simulink model "AXI_QPSK_Tx"  (R2023b)
settings: Solver=FixedStepAuto  StartTime=0.0  StopTime=10/Rb  RelTol=1e-3
PreLoadFcn:
  | Rb = 1000;   % 1kbit / s
  | Rsym = Rb/2;   % 2 bits per symbol
  | Rsymbol = Rb/2;
  | OSR = 32;
  | f_error = 120;
  | 
  | design_filters_tx
values from neighbouring files (symbols this model uses):
  CIC_fine_Tx = 2^-(CIC_right_shift - CIC_left_shift - CIC_shift_Tx)    [design_filters_tx.m]
  fCIC = fCICcomp * R_CIC    (= 25600000)    [design_filters_tx.m]
  fHB = fRRC * R_HB    (= 4000)    [design_filters_tx.m]
  R_CIC = 3200    [design_filters_tx.m]
  R_CICcomp = 2    [design_filters_tx.m]
  R_HB = 2    [design_filters_tx.m]
  R_RRC = 4    [design_filters_tx.m]
undefined symbols (not defined in the file or in its folder): AXI4, Lite
libraries: hdlBasic x309, hdlDSPIP x8, hdlsllib x2, vmcUtilities x1
(part 3 of 3)

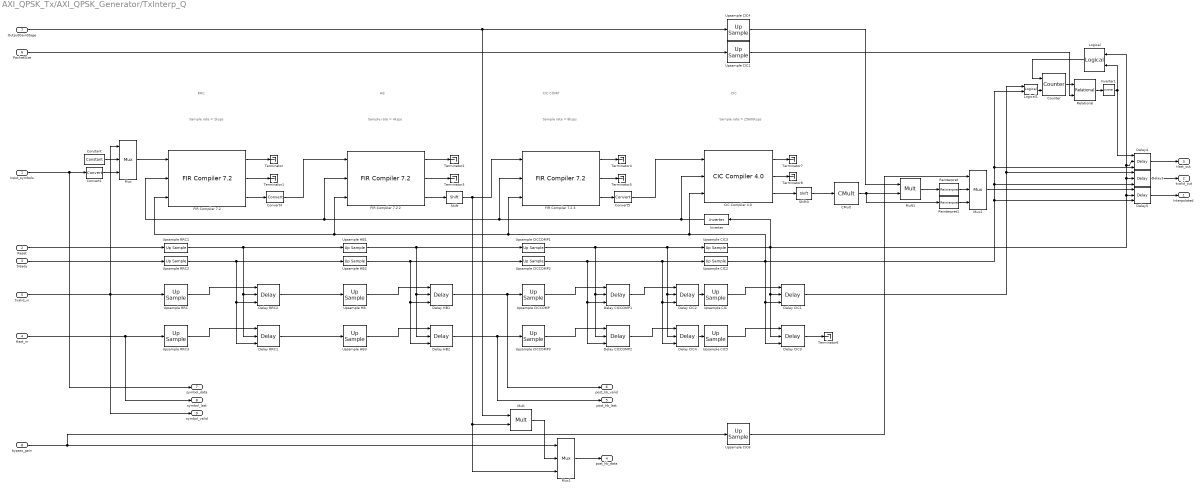
== system AXI_QPSK_Tx/AXI_QPSK_Generator/TxInterp_Q ==
  note: Sample rate
      | = 25600ksps
  note: Sample rate
      | = 8ksps
  note: Sample rate
      | = 4ksps
  note: Sample rate
      | = 2ksps
  note: CIC
  note: CIC COMP
  note: RRC
  note: HB
  Input_symbols : Inport
  Reset : Inport  Port=2
  tready : Inport  Port=3
  tlast_in : Inport  Port=4
  tvalid_in : Inport  Port=5
  PacketSize : Inport  Port=6
  OutputGainStage : Inport  Port=7
  bypass_gain : Inport  Port=8
  "CIC Compiler 4.0 " : hdlDSPIP/CIC Compiler 4.0   filter_type=Interpolation  number_of_stages=5  differential_delay=1  number_of_channels=1  sample_rate_changes=Fixed  fixed_or_initial_rate=R_CIC  minimum_rate=3200  maximum_rate=3200  ratespecification=Maximum_Possible  sampleperiod=3200  hardwareoversamplingrate=1  quantization=Full_Precision  output_data_width=65  use_xtreme_dsp_slice=on  use_streaming_interface=on  has_aclken=on  has_aresetn=on  has_dout_tready=off  trim_axipin_name=on  gui_behaviour=Sysgen_GUI  input_data_width=18  ip_name=CIC Compiler  ip_version=4.0  dsptool_ready=true  wrapper_available=true  port_translation_map={ 'aclken' => 'en', 'aresetn' => 'rst' }  ipcore_xco_need_fpga_part=true  ipcore_fpga_part=[]  ipcore_verbose=false  XmcBlockStatus=1  maskContainerNames=tabcontainer1  block_type=cic_compiler_v4_0  block_config=sysgen:rodinimport_config
  CMult : hdlBasic/CMult  const=CIC_fine_Tx  gui_display_data_type=Fixed-point  const_n_bits=16  const_bin_pt=15  float_type=Single  exp_bits=8  fraction_bits=24  en=off  latency=0  precision=User Defined  arith_type="Signed  (2's comp)"  n_bits=16  bin_pt=15  quantization=Truncate  overflow=Wrap  use_behavioral_HDL=off  mem_type=Distributed RAM  pipeline=off  XmcBlockStatus=1  maskContainerNames=tabcontainer1  block_type=cmult  block_config=sysgen:CMult_config
      settings: infoedit=[]
  Constant : hdlBasic/Constant  const=0  gui_display_data_type=Fixed-point  arith_type=Signed (2's comp)  n_bits=16  bin_pt=0  preci_type=Single  exp_width=8  frac_width=24  explicit_period=on  period=2/Rb  XmcBlockStatus=1  maskContainerNames=tabcontainer1  block_type=constant  block_config=sysgen:Constant_config
  Convert1 : hdlBasic/Convert  gui_display_data_type=Fixed-point  arith_type="Signed  (2's comp)"  n_bits=16  bin_pt=0  float_type=Single  exp_bits=8  fraction_bits=24  quantization=Truncate  overflow=Wrap  en=off  latency=0  pipeline=off  XmcBlockStatus=1  maskContainerNames=group2  block_type=convert  block_config=sysgen:Convert_config  block_width=595  block_height=885
  Convert4 : hdlBasic/Convert  gui_display_data_type=Fixed-point  arith_type="Signed  (2's comp)"  n_bits=16  bin_pt=15  float_type=Single  exp_bits=8  fraction_bits=24  quantization=Truncate  overflow=Wrap  en=off  latency=0  pipeline=off  XmcBlockStatus=1  maskContainerNames=group2  block_type=convert  block_config=sysgen:Convert_config  block_width=595  block_height=885
  Convert5 : hdlBasic/Convert  gui_display_data_type=Fixed-point  arith_type="Signed  (2's comp)"  n_bits=16  bin_pt=15  float_type=Single  exp_bits=8  fraction_bits=24  quantization=Truncate  overflow=Wrap  en=off  latency=0  pipeline=off  XmcBlockStatus=1  maskContainerNames=group2  block_type=convert  block_config=sysgen:Convert_config  block_width=595  block_height=885
  Counter : hdlBasic/Counter  cnt_type=Free running  cnt_to=Inf  operation=Up  start_count=0  cnt_by_val=1  arith_type=Unsigned  n_bits=32  bin_pt=0  load_pin=off  rst=on  en=on  explicit_period=Explicit  period=1/fCIC  use_behavioral_HDL=off  implementation=Fabric  XmcBlockStatus=1  maskContainerNames=group1  block_type=counter  block_config=sysgen:Counter_config  block_width=531  block_height=1023
  Delay CIC1 : hdlBasic/Delay  rst=on  en=on  latency=3*8  reg_retiming=off  XmcBlockStatus=1  maskContainerNames=group1  block_type=delay  block_config=sysgen:Delay_config
  Delay CIC2 : hdlBasic/Delay  rst=on  en=on  latency=4  reg_retiming=off  XmcBlockStatus=1  maskContainerNames=group1  block_type=delay  block_config=sysgen:Delay_config
  Delay CIC3 : hdlBasic/Delay  rst=on  en=on  latency=3*8-1  reg_retiming=off  XmcBlockStatus=1  maskContainerNames=group1  block_type=delay  block_config=sysgen:Delay_config
  Delay CIC4 : hdlBasic/Delay  rst=on  en=on  latency=5  reg_retiming=off  XmcBlockStatus=1  maskContainerNames=group1  block_type=delay  block_config=sysgen:Delay_config
  Delay CICCOMP1 : hdlBasic/Delay  rst=on  en=on  latency=R_CICcomp*4  reg_retiming=off  XmcBlockStatus=1  maskContainerNames=group1  block_type=delay  block_config=sysgen:Delay_config
  Delay CICCOMP2 : hdlBasic/Delay  rst=on  en=on  latency=R_CICcomp*4+1  reg_retiming=off  XmcBlockStatus=1  maskContainerNames=group1  block_type=delay  block_config=sysgen:Delay_config
  Delay HB1 : hdlBasic/Delay  rst=on  en=on  latency=R_HB*2  reg_retiming=off  XmcBlockStatus=1  maskContainerNames=group1  block_type=delay  block_config=sysgen:Delay_config
  Delay HB2 : hdlBasic/Delay  rst=on  en=on  latency=R_HB*2+1  reg_retiming=off  XmcBlockStatus=1  maskContainerNames=group1  block_type=delay  block_config=sysgen:Delay_config
  Delay RRC1 : hdlBasic/Delay  rst=on  en=on  latency=3*R_RRC  reg_retiming=off  XmcBlockStatus=1  maskContainerNames=group1  block_type=delay  block_config=sysgen:Delay_config
  Delay RRC2 : hdlBasic/Delay  rst=on  en=on  latency=R_RRC*2+1  reg_retiming=off  XmcBlockStatus=1  maskContainerNames=group1  block_type=delay  block_config=sysgen:Delay_config
  Delay3 : hdlBasic/Delay  rst=on  en=on  latency=1  reg_retiming=off  XmcBlockStatus=1  maskContainerNames=group1  block_type=delay  block_config=sysgen:Delay_config
  Delay4 : hdlBasic/Delay  rst=on  en=on  latency=1  reg_retiming=off  XmcBlockStatus=1  maskContainerNames=group1  block_type=delay  block_config=sysgen:Delay_config
  Delay5 : hdlBasic/Delay  rst=on  en=on  latency=1  reg_retiming=off  XmcBlockStatus=1  maskContainerNames=group1  block_type=delay  block_config=sysgen:Delay_config
  "FIR Compiler 7.2 " : hdlDSPIP/FIR Compiler 7.2   coefficientvector=WRRC.Numerator  coefficient_sets=1  coefficient_reload=off  filter_type=Interpolation  rate_change_type=Integer  interpolation_rate=R_RRC  decimation_rate=1  zero_pack_factor=1  channel_sequence=Basic  number_channels=1  pattern_list='P4-0,P4-1,P4-2,P4-3,P4-4'  number_paths=1  ratespecification=Maximum_Possible  sampleperiod=1  hardwareoversamplingrate=1  coefficient_sign=Signed  quantization=Quantize_Only  coefficient_width=16  bestprecision=on  coefficient_fractional_bits=15  coefficient_structure=Inferred  output_rounding_mode=Full_Precision  output_width=31  filter_architecture=Systolic_Multiply_Accumulate  optimization_goal=Area  optimization_list='None'  data_buffer_type=Automatic  coefficient_buffer_type=Automatic  input_buffer_type=Automatic  output_buffer_type=Automatic  preference_for_other_storage=Automatic  multi_column_support=Automatic  columnconfig='13'  inter_column_pipe_length=4  data_has_tlast=Not_Required  m_data_has_tready=off  s_data_has_fifo=off  s_data_has_tuser=Not_Required  m_data_has_tuser=Not_Required  s_config_sync_mode=On_Vector  s_config_method=Single  num_reload_slots=1  has_aclken=on  has_aresetn=on  reset_data_vector=on  trim_axipin_name=on  simulation_type=hybrid_sim  simulation_model=sysgen:xfirv7_2_cmodel  data_path_portlist={ 's_axis_data_tdata', 'm_axis_data_tdata' }  passband_min=0.0  passband_max=0.5  stopband_min=0.5  stopband_max=1.0  filter_selection=1  gui_behaviour='Sysgen_GUI'  data_sign=Signed  data_width=16  data_fractional_bits=0  data_tuser_width=1  wrapper_available=true  ip_wrap_arbitrary_binary_point=true  ip_name=FIR Compiler  ip_version=7.2  dsptool_ready=true  ipcore_usecache=true  ipcore_useipmodelcache=true  port_translation_map={ 'aclken' => 'en', 'aresetn' => 'rst' }  run_core_at_system_period=true  ipcore_xco_need_fpga_part=true  ipcore_fpga_part=[]  XmcBlockStatus=1  maskContainerNames=tabcontainer1  block_type=fir_compiler_v7_2  block_config=sysgen:rodinimport_config  block_width=820  block_height=600
  FIR Compiler 7.2 2 : hdlDSPIP/FIR Compiler 7.2   coefficientvector=HB.Numerator  coefficient_sets=1  coefficient_reload=off  filter_type=Interpolation  rate_change_type=Integer  interpolation_rate=2  decimation_rate=1  zero_pack_factor=1  channel_sequence=Basic  number_channels=1  pattern_list='P4-0,P4-1,P4-2,P4-3,P4-4'  number_paths=1  ratespecification=Maximum_Possible  sampleperiod=1  hardwareoversamplingrate=1  coefficient_sign=Signed  quantization=Quantize_Only  coefficient_width=16  bestprecision=on  coefficient_fractional_bits=15  coefficient_structure=Inferred  output_rounding_mode=Full_Precision  output_width=32  filter_architecture=Systolic_Multiply_Accumulate  optimization_goal=Area  optimization_list='None'  data_buffer_type=Automatic  coefficient_buffer_type=Automatic  input_buffer_type=Automatic  output_buffer_type=Automatic  preference_for_other_storage=Automatic  multi_column_support=Automatic  columnconfig='6'  inter_column_pipe_length=4  data_has_tlast=Not_Required  m_data_has_tready=off  s_data_has_fifo=off  s_data_has_tuser=Not_Required  m_data_has_tuser=Not_Required  s_config_sync_mode=On_Vector  s_config_method=Single  num_reload_slots=1  has_aclken=on  has_aresetn=on  reset_data_vector=on  trim_axipin_name=on  simulation_type=hybrid_sim  simulation_model=sysgen:xfirv7_2_cmodel  data_path_portlist={ 's_axis_data_tdata', 'm_axis_data_tdata' }  passband_min=0.0  passband_max=0.5  stopband_min=0.5  stopband_max=1.0  filter_selection=1  gui_behaviour='Sysgen_GUI'  data_sign=Signed  data_width=16  data_fractional_bits=0  data_tuser_width=1  wrapper_available=true  ip_wrap_arbitrary_binary_point=true  ip_name=FIR Compiler  ip_version=7.2  dsptool_ready=true  ipcore_usecache=true  ipcore_useipmodelcache=true  port_translation_map={ 'aclken' => 'en', 'aresetn' => 'rst' }  run_core_at_system_period=true  ipcore_xco_need_fpga_part=true  ipcore_fpga_part=[]  XmcBlockStatus=1  maskContainerNames=tabcontainer1  block_type=fir_compiler_v7_2  block_config=sysgen:rodinimport_config  block_width=820  block_height=600
  FIR Compiler 7.2 3 : hdlDSPIP/FIR Compiler 7.2   coefficientvector=WComp.Numerator  coefficient_sets=1  coefficient_reload=off  filter_type=Interpolation  rate_change_type=Integer  interpolation_rate=R_CICcomp  decimation_rate=1  zero_pack_factor=1  channel_sequence=Basic  number_channels=1  pattern_list='P4-0,P4-1,P4-2,P4-3,P4-4'  number_paths=1  ratespecification=Maximum_Possible  sampleperiod=1  hardwareoversamplingrate=1  coefficient_sign=Signed  quantization=Quantize_Only  coefficient_width=16  bestprecision=on  coefficient_fractional_bits=15  coefficient_structure=Inferred  output_rounding_mode=Full_Precision  output_width=33  filter_architecture=Systolic_Multiply_Accumulate  optimization_goal=Area  optimization_list='None'  data_buffer_type=Automatic  coefficient_buffer_type=Automatic  input_buffer_type=Automatic  output_buffer_type=Automatic  preference_for_other_storage=Automatic  multi_column_support=Automatic  columnconfig='19'  inter_column_pipe_length=4  data_has_tlast=Not_Required  m_data_has_tready=off  s_data_has_fifo=off  s_data_has_tuser=Not_Required  m_data_has_tuser=Not_Required  s_config_sync_mode=On_Vector  s_config_method=Single  num_reload_slots=1  has_aclken=on  has_aresetn=on  reset_data_vector=on  trim_axipin_name=on  simulation_type=hybrid_sim  simulation_model=sysgen:xfirv7_2_cmodel  data_path_portlist={ 's_axis_data_tdata', 'm_axis_data_tdata' }  passband_min=0.0  passband_max=0.5  stopband_min=0.5  stopband_max=1.0  filter_selection=1  gui_behaviour='Sysgen_GUI'  data_sign=Signed  data_width=16  data_fractional_bits=0  data_tuser_width=1  wrapper_available=true  ip_wrap_arbitrary_binary_point=true  ip_name=FIR Compiler  ip_version=7.2  dsptool_ready=true  ipcore_usecache=true  ipcore_useipmodelcache=true  port_translation_map={ 'aclken' => 'en', 'aresetn' => 'rst' }  run_core_at_system_period=true  ipcore_xco_need_fpga_part=true  ipcore_fpga_part=[]  XmcBlockStatus=1  maskContainerNames=tabcontainer1  block_type=fir_compiler_v7_2  block_config=sysgen:rodinimport_config  block_width=820  block_height=600
  Inverter : hdlBasic/Inverter  en=off  latency=0  XmcBlockStatus=1  maskContainerNames=group2  block_type=inv  block_config=sysgen:Inverter_config
  Inverter1 : hdlBasic/Inverter  en=off  latency=0  XmcBlockStatus=1  maskContainerNames=group2  block_type=inv  block_config=sysgen:Inverter_config
  Logical : hdlBasic/Logical  logical_function=OR  inputs=2  en=off  latency=0  precision=Full  arith_type=Unsigned  n_bits=16  bin_pt=0  align_bp=on  overflow=[]  quantization=[]  XmcBlockStatus=1  maskContainerNames=tabcontainer1  block_type=logical  block_config=sysgen:Logical_config
  Logical1 : hdlBasic/Logical  logical_function=AND  inputs=2  en=off  latency=0  precision=Full  arith_type=Unsigned  n_bits=16  bin_pt=0  align_bp=on  overflow=[]  quantization=[]  XmcBlockStatus=1  maskContainerNames=tabcontainer1  block_type=logical  block_config=sysgen:Logical_config
  Mult : hdlBasic/Mult  precision=User Defined  arith_type="Signed  (2's comp)"  n_bits=16  bin_pt=15  quantization=Truncate  overflow=Wrap  en=off  latency=0  use_behavioral_HDL=off  opt=Speed  use_embedded=on  optimum_pipeline=off  pipeline=on  use_rpm=on  placement_style=Triangular  XmcBlockStatus=1  maskContainerNames=group1  block_type=mult  block_config=sysgen:Mult_config  block_width=598  block_height=876
  Mult1 : hdlBasic/Mult  precision=User Defined  arith_type="Signed  (2's comp)"  n_bits=16  bin_pt=15  quantization=Truncate  overflow=Wrap  en=off  latency=0  use_behavioral_HDL=off  opt=Speed  use_embedded=on  optimum_pipeline=off  pipeline=on  use_rpm=on  placement_style=Triangular  XmcBlockStatus=1  maskContainerNames=group1  block_type=mult  block_config=sysgen:Mult_config  block_width=598  block_height=876
  Mux : hdlBasic/Mux  inputs=2  en=off  latency=0  precision=Full  arith_type=Unsigned  n_bits=16  bin_pt=14  quantization=Truncate  overflow=Wrap  XmcBlockStatus=1  maskContainerNames=tabcontainer1  block_type=mux  block_config=sysgen:Mux_config
  Mux1 : hdlBasic/Mux  inputs=2  en=off  latency=0  precision=Full  arith_type=Unsigned  n_bits=16  bin_pt=14  quantization=Truncate  overflow=Wrap  XmcBlockStatus=1  maskContainerNames=tabcontainer1  block_type=mux  block_config=sysgen:Mux_config
  Mux2 : hdlBasic/Mux  inputs=2  en=off  latency=0  precision=Full  arith_type=Unsigned  n_bits=16  bin_pt=14  quantization=Truncate  overflow=Wrap  XmcBlockStatus=1  maskContainerNames=tabcontainer1  block_type=mux  block_config=sysgen:Mux_config
  Reinterpret : hdlBasic/Reinterpret  force_arith_type=on  arith_type=Unsigned  force_bin_pt=on  bin_pt=0  XmcBlockStatus=1  maskContainerNames=group1  block_type=reinterpret  block_config=sysgen:Reinterpret_config
  Reinterpret1 : hdlBasic/Reinterpret  force_arith_type=on  arith_type=Unsigned  force_bin_pt=on  bin_pt=0  XmcBlockStatus=1  maskContainerNames=group1  block_type=reinterpret  block_config=sysgen:Reinterpret_config
  Relational : hdlBasic/Relational  mode=a<b  op_type=Bool  en=off  latency=0  XmcBlockStatus=1  maskContainerNames=tabcontainer1  block_type=relational  block_config=sysgen:Relational_config
  Shift : hdlBasic/Shift  shift_dir=Left  shift_bits=1  en=off  latency=0  precision=User Defined  arith_type="Signed  (2's comp)"  n_bits=16  bin_pt=15  quantization=Truncate  overflow=Wrap  XmcBlockStatus=1  maskContainerNames=group2  block_type=shift  block_config=sysgen:Shift_config
  Shift3 : hdlBasic/Shift  shift_dir=Right  shift_bits=CIC_shift_Tx  en=off  latency=0  precision=User Defined  arith_type="Signed  (2's comp)"  n_bits=17  bin_pt=14  quantization=Truncate  overflow=Wrap  XmcBlockStatus=1  maskContainerNames=group2  block_type=shift  block_config=sysgen:Shift_config
  Terminator{,1..8} (9 alike) : Terminator
  Upsample CIC : hdlBasic/Up Sample  sample_ratio=R_CIC  copy_samples=on  en=off  latency=0  XmcBlockStatus=1  maskContainerNames=group1  block_type=usamp  block_config=sysgen:Upsample_config
  Upsample CIC1 : hdlBasic/Up Sample  sample_ratio=fCIC/(Rb/2)  copy_samples=on  en=off  latency=0  XmcBlockStatus=1  maskContainerNames=group1  block_type=usamp  block_config=sysgen:Upsample_config
  Upsample CIC2 : hdlBasic/Up Sample  sample_ratio=R_CIC  copy_samples=on  en=off  latency=0  XmcBlockStatus=1  maskContainerNames=group1  block_type=usamp  block_config=sysgen:Upsample_config
  Upsample CIC3 : hdlBasic/Up Sample  sample_ratio=R_CIC  copy_samples=on  en=off  latency=0  XmcBlockStatus=1  maskContainerNames=group1  block_type=usamp  block_config=sysgen:Upsample_config
  Upsample CIC4 : hdlBasic/Up Sample  sample_ratio=fCIC/fHB  copy_samples=on  en=off  latency=0  XmcBlockStatus=1  maskContainerNames=group1  block_type=usamp  block_config=sysgen:Upsample_config
  Upsample CIC5 : hdlBasic/Up Sample  sample_ratio=R_CIC  copy_samples=off  en=off  latency=0  XmcBlockStatus=1  maskContainerNames=group1  block_type=usamp  block_config=sysgen:Upsample_config
  Upsample CIC6 : hdlBasic/Up Sample  sample_ratio=fCIC/fHB  copy_samples=on  en=off  latency=0  XmcBlockStatus=1  maskContainerNames=group1  block_type=usamp  block_config=sysgen:Upsample_config
  Upsample CICCOMP : hdlBasic/Up Sample  sample_ratio=R_CICcomp  copy_samples=on  en=off  latency=0  XmcBlockStatus=1  maskContainerNames=group1  block_type=usamp  block_config=sysgen:Upsample_config
  Upsample CICCOMP1 : hdlBasic/Up Sample  sample_ratio=R_CICcomp  copy_samples=on  en=off  latency=0  XmcBlockStatus=1  maskContainerNames=group1  block_type=usamp  block_config=sysgen:Upsample_config
  Upsample CICCOMP2 : hdlBasic/Up Sample  sample_ratio=R_CICcomp  copy_samples=on  en=off  latency=0  XmcBlockStatus=1  maskContainerNames=group1  block_type=usamp  block_config=sysgen:Upsample_config
  Upsample CICCOMP3 : hdlBasic/Up Sample  sample_ratio=R_CICcomp  copy_samples=off  en=off  latency=0  XmcBlockStatus=1  maskContainerNames=group1  block_type=usamp  block_config=sysgen:Upsample_config
  Upsample HB : hdlBasic/Up Sample  sample_ratio=R_HB  copy_samples=on  en=off  latency=0  XmcBlockStatus=1  maskContainerNames=group1  block_type=usamp  block_config=sysgen:Upsample_config
  Upsample HB1 : hdlBasic/Up Sample  sample_ratio=R_HB  copy_samples=on  en=off  latency=0  XmcBlockStatus=1  maskContainerNames=group1  block_type=usamp  block_config=sysgen:Upsample_config
  Upsample HB2 : hdlBasic/Up Sample  sample_ratio=R_HB  copy_samples=on  en=off  latency=0  XmcBlockStatus=1  maskContainerNames=group1  block_type=usamp  block_config=sysgen:Upsample_config
  Upsample HB3 : hdlBasic/Up Sample  sample_ratio=R_HB  copy_samples=off  en=off  latency=0  XmcBlockStatus=1  maskContainerNames=group1  block_type=usamp  block_config=sysgen:Upsample_config
  Upsample RRC : hdlBasic/Up Sample  sample_ratio=R_RRC  copy_samples=on  en=off  latency=0  XmcBlockStatus=1  maskContainerNames=group1  block_type=usamp  block_config=sysgen:Upsample_config
  Upsample RRC1 : hdlBasic/Up Sample  sample_ratio=R_RRC  copy_samples=on  en=off  latency=0  XmcBlockStatus=1  maskContainerNames=group1  block_type=usamp  block_config=sysgen:Upsample_config
  Upsample RRC2 : hdlBasic/Up Sample  sample_ratio=R_RRC  copy_samples=on  en=off  latency=0  XmcBlockStatus=1  maskContainerNames=group1  block_type=usamp  block_config=sysgen:Upsample_config
  Upsample RRC3 : hdlBasic/Up Sample  sample_ratio=R_RRC  copy_samples=off  en=off  latency=0  XmcBlockStatus=1  maskContainerNames=group1  block_type=usamp  block_config=sysgen:Upsample_config
  Interpolated : Outport  VectorParamsAs1DForOutWhenUnconnected=off
  tvalid_out : Outport  Port=2  VectorParamsAs1DForOutWhenUnconnected=off
  tlast_out : Outport  Port=3  VectorParamsAs1DForOutWhenUnconnected=off
  post_hb_data : Outport  Port=4  VectorParamsAs1DForOutWhenUnconnected=off
  post_hb_last : Outport  Port=5  VectorParamsAs1DForOutWhenUnconnected=off
  post_hb_valid : Outport  Port=6  VectorParamsAs1DForOutWhenUnconnected=off
  symbol_data : Outport  Port=7  VectorParamsAs1DForOutWhenUnconnected=off
  symbol_last : Outport  Port=8  VectorParamsAs1DForOutWhenUnconnected=off
  symbol_valid : Outport  Port=9  VectorParamsAs1DForOutWhenUnconnected=off
  wires:
  Mult/1 -> Mux1/2
  Mux1/1 -> post_hb_data/1
  Upsample CIC4/1 -> Mult1/1
  Mult1/1 -> Reinterpret/1
  Delay CIC3/1 -> Terminator6/1
  Delay HB1/1 -> Upsample CICCOMP/1, post_hb_valid/1
  Delay HB2/1 -> post_hb_last/1, Upsample CICCOMP3/1
  Constant/1 -> Mux/2
  Input_symbols/1 -> symbol_data/1, Convert1/1
  Mux/1 -> "FIR Compiler 7.2 "/1
  Delay CICCOMP2/1 -> Delay CIC4/1
  Delay CIC4/1 -> Upsample CIC5/1
  Delay CICCOMP1/1 -> Delay CIC2/1
  Delay CIC2/1 -> Upsample CIC/1
  Inverter/1 -> "CIC Compiler 4.0 "/2, FIR Compiler 7.2 2/2, "FIR Compiler 7.2 "/2, FIR Compiler 7.2 3/2
  Upsample CIC5/1 -> Delay CIC3/1
  Upsample RRC1/1 -> Upsample HB1/1, Delay RRC2/2, Delay RRC1/2
  Upsample RRC2/1 -> Upsample HB2/1, Delay RRC2/3, Delay RRC1/3
  Upsample HB1/1 -> Upsample CICCOMP1/1, Delay HB1/2, Delay HB2/2
  Upsample HB2/1 -> Upsample CICCOMP2/1, Delay HB1/3, Delay HB2/3
  Upsample CICCOMP1/1 -> Upsample CIC3/1, Delay CIC2/2, Delay CIC4/2, Delay CICCOMP1/2, Delay CICCOMP2/2
  Upsample CICCOMP2/1 -> Upsample CIC2/1, Delay CIC2/3, Delay CIC4/3, Delay CICCOMP1/3, Delay CICCOMP2/3
  tlast_in/1 -> symbol_last/1, Upsample RRC3/1
  Delay RRC1/1 -> Upsample HB3/1
  Upsample RRC3/1 -> Delay RRC1/1
  Upsample HB3/1 -> Delay HB2/1
  Upsample CICCOMP3/1 -> Delay CICCOMP2/1
  tready/1 -> Upsample RRC2/1
  Delay CIC1/1 -> Delay3/1, Logical1/1
  Upsample CICCOMP/1 -> Delay CICCOMP1/1
  Upsample HB/1 -> Delay HB1/1
  Upsample RRC/1 -> Delay RRC2/1
  Delay RRC2/1 -> Upsample HB/1
  tvalid_in/1 -> Mux/1, symbol_valid/1, Upsample RRC/1
  Upsample CIC3/1 -> Inverter/1, Delay4/2, Logical/1, Delay3/2, Delay5/2, Delay CIC1/2, Delay CIC3/2
  Upsample CIC2/1 -> "CIC Compiler 4.0 "/3, FIR Compiler 7.2 3/3, FIR Compiler 7.2 2/3, "FIR Compiler 7.2 "/3, Delay5/3, Delay3/3, Delay4/3, Logical1/2, Delay CIC1/3, Delay CIC3/3
  "CIC Compiler 4.0 "/2 -> Terminator8/1
  Upsample CIC/1 -> Delay CIC1/1
  Reset/1 -> Upsample RRC1/1
  Convert5/1 -> "CIC Compiler 4.0 "/1
  "CIC Compiler 4.0 "/1 -> Terminator7/1
  FIR Compiler 7.2 3/2 -> Terminator5/1
  FIR Compiler 7.2 3/1 -> Terminator4/1
  FIR Compiler 7.2 3/3 -> Convert5/1
  FIR Compiler 7.2 2/1 -> Terminator2/1
  FIR Compiler 7.2 2/2 -> Terminator3/1
  FIR Compiler 7.2 2/3 -> Shift/1
  "FIR Compiler 7.2 "/3 -> Convert4/1
  Shift3/1 -> CMult/1
  "FIR Compiler 7.2 "/2 -> Terminator1/1
  "FIR Compiler 7.2 "/1 -> Terminator/1
  PacketSize/1 -> Upsample CIC1/1
  Upsample CIC1/1 -> Relational/2
  Counter/1 -> Relational/1
  Logical/1 -> Counter/1
  Inverter1/1 -> Delay4/1, Logical/2
  Relational/1 -> Inverter1/1
  Delay4/1 -> tlast_out/1
  Delay3/1 -> tvalid_out/1
  Delay5/1 -> Interpolated/1
  Logical1/1 -> Counter/2
  "CIC Compiler 4.0 "/3 -> Shift3/1
  Convert4/1 -> FIR Compiler 7.2 2/1
  Convert1/1 -> Mux/3
  Shift/1 -> FIR Compiler 7.2 3/1, Mult/2, Mux1/3
  CMult/1 -> Mult1/2, Reinterpret1/1
  OutputGainStage/1 -> Upsample CIC4/1, Mult/1
  Reinterpret/1 -> Mux2/2
  Mux2/1 -> Delay5/1
  Reinterpret1/1 -> Mux2/3
  bypass_gain/1 -> Upsample CIC6/1, Mux1/1
  Upsample CIC6/1 -> Mux2/1

== system AXI_QPSK_Tx/AXI_QPSK_Generator/PostHB_Time_Domain/M_AXIS_SYMBOL_CTRL ==
  i_data : Inport
  tvalid_in : Inport  Port=2
  q_data : Inport  Port=3
  reset : Inport  Port=4
  packet_size : Inport  Port=5
  tready_in : Inport  Port=6
  transfer : Inport  Port=7
  auto_restart : Inport  Port=8
  AXI_Write_Interface : Subsystem
  Concat : hdlBasic/Concat  num_inputs=2  XmcBlockStatus=1  maskContainerNames=group1  block_type=concat  block_config=sysgen:Concat_config
  Reinterpret : hdlBasic/Reinterpret  force_arith_type=on  arith_type=Unsigned  force_bin_pt=on  bin_pt=0  XmcBlockStatus=1  maskContainerNames=group1  block_type=reinterpret  block_config=sysgen:Reinterpret_config
  Reinterpret1 : hdlBasic/Reinterpret  force_arith_type=on  arith_type=Unsigned  force_bin_pt=on  bin_pt=0  XmcBlockStatus=1  maskContainerNames=group1  block_type=reinterpret  block_config=sysgen:Reinterpret_config
  tdata_out : Outport  VectorParamsAs1DForOutWhenUnconnected=off
  tvalid_out : Outport  Port=2  VectorParamsAs1DForOutWhenUnconnected=off
  tlast_out : Outport  Port=3  VectorParamsAs1DForOutWhenUnconnected=off
  wires:
  AXI_Write_Interface/1(tdata_out) -> tdata_out/1
  AXI_Write_Interface/3(tvalid_out) -> tvalid_out/1
  AXI_Write_Interface/2(tlast_out) -> tlast_out/1
  tready_in/1 -> AXI_Write_Interface/7(tready)
  auto_restart/1 -> AXI_Write_Interface/3(auto_restart)
  transfer/1 -> AXI_Write_Interface/2(transfer)
  Concat/1 -> AXI_Write_Interface/5(tdata_in)
  reset/1 -> AXI_Write_Interface/1(int_reset)
  tvalid_in/1 -> AXI_Write_Interface/6(tvalid_in)
  packet_size/1 -> AXI_Write_Interface/4(packet_size)
  Reinterpret/1 -> Concat/1
  Reinterpret1/1 -> Concat/2
  q_data/1 -> Reinterpret/1
  i_data/1 -> Reinterpret1/1

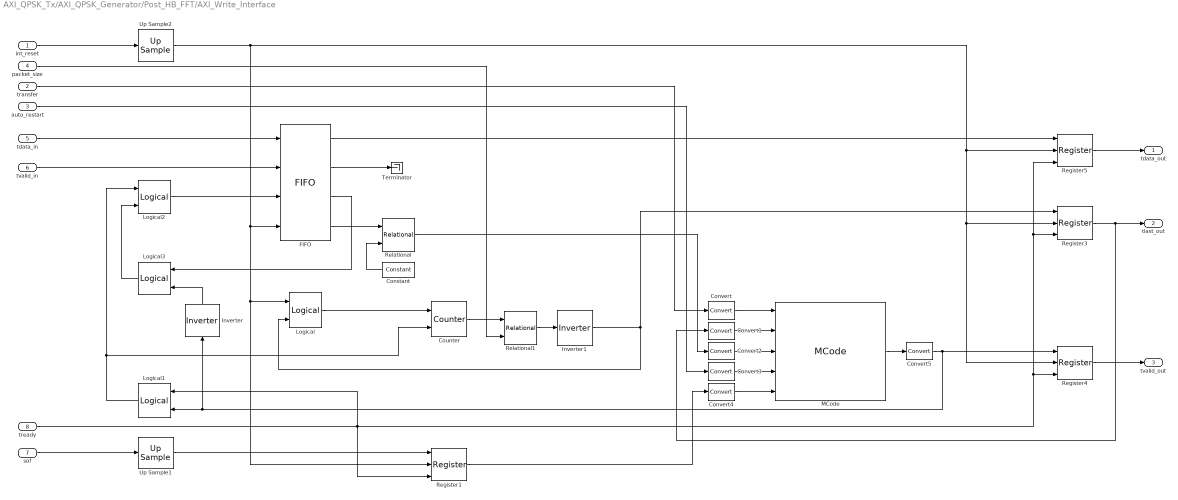
== system AXI_QPSK_Tx/AXI_QPSK_Generator/Post_HB_FFT/AXI_Write_Interface ==
  int_reset : Inport
  transfer : Inport  Port=2
  auto_restart : Inport  Port=3
  packet_size : Inport  Port=4
  tdata_in : Inport  Port=5
  tvalid_in : Inport  Port=6
  sof : Inport  Port=7
  tready : Inport  Port=8
  Constant : hdlBasic/Constant  const=8192/2-1  gui_display_data_type=Fixed-point  arith_type=Unsigned  n_bits=13  bin_pt=0  preci_type=Single  exp_width=8  frac_width=24  explicit_period=on  period=1/fCIC  XmcBlockStatus=1  maskContainerNames=tabcontainer1  block_type=constant  block_config=sysgen:Constant_config
  Convert{,1..4} (5 alike) : hdlBasic/Convert  gui_display_data_type=Fixed-point  arith_type=Unsigned  n_bits=1  bin_pt=0  float_type=Single  exp_bits=8  fraction_bits=24  quantization=Truncate  overflow=Wrap  en=off  latency=0  pipeline=off  XmcBlockStatus=1  maskContainerNames=group2  block_type=convert  block_config=sysgen:Convert_config  block_width=595  block_height=885
  Convert5 : hdlBasic/Convert  gui_display_data_type=Boolean  arith_type=Boolean  n_bits=1  bin_pt=0  float_type=Single  exp_bits=8  fraction_bits=24  quantization=Truncate  overflow=Wrap  en=off  latency=0  pipeline=off  XmcBlockStatus=1  maskContainerNames=group2  block_type=convert  block_config=sysgen:Convert_config  block_width=595  block_height=885
  Counter : hdlBasic/Counter  cnt_type=Free running  cnt_to=Inf  operation=Up  start_count=0  cnt_by_val=1  arith_type=Unsigned  n_bits=32  bin_pt=0  load_pin=off  rst=on  en=on  explicit_period=Explicit  period=1/fCIC  use_behavioral_HDL=off  implementation=Fabric  XmcBlockStatus=1  maskContainerNames=group1  block_type=counter  block_config=sysgen:Counter_config  block_width=531  block_height=1023
  FIFO : hdlBasic/FIFO  mem_type=Block RAM  performance_options=Standard_FIFO  embedded_registers=off  depth=8K  use_asym_data_widths=off  asym_read_width=32  percent_nbits=1  rst=on  rst_latency=2  en=off  use_dcount=on  use_percent_full_port=off  use_almost_empty=off  almost_empty_thresh=2  use_almost_full=off  use_rd_rst_busy=off  use_wr_rst_busy=off  almost_full_thresh=14  almost_empty_offset=[]  almost_full_offset=[]  explicit_period=off  period=[]  store_only_valid=[]  init_zero=[]  simulation_type=fast_sim  XmcBlockStatus=1  maskContainerNames=tabcontainer1  block_type=fifo  block_config=sysgen:FIFO_config  block_width=538  block_height=997
      settings: infoedit=[]
  Inverter : hdlBasic/Inverter  en=off  latency=0  XmcBlockStatus=1  maskContainerNames=group2  block_type=inv  block_config=sysgen:Inverter_config
  Inverter1 : hdlBasic/Inverter  en=off  latency=0  XmcBlockStatus=1  maskContainerNames=group2  block_type=inv  block_config=sysgen:Inverter_config
  Logical : hdlBasic/Logical  logical_function=OR  inputs=2  en=off  latency=0  precision=Full  arith_type=Unsigned  n_bits=16  bin_pt=0  align_bp=on  overflow=[]  quantization=[]  XmcBlockStatus=1  maskContainerNames=tabcontainer1  block_type=logical  block_config=sysgen:Logical_config
  Logical1 : hdlBasic/Logical  logical_function=AND  inputs=2  en=off  latency=0  precision=Full  arith_type=Unsigned  n_bits=16  bin_pt=0  align_bp=on  overflow=[]  quantization=[]  XmcBlockStatus=1  maskContainerNames=tabcontainer1  block_type=logical  block_config=sysgen:Logical_config
  Logical2 : hdlBasic/Logical  logical_function=OR  inputs=2  en=off  latency=0  precision=Full  arith_type=Unsigned  n_bits=16  bin_pt=0  align_bp=on  overflow=[]  quantization=[]  XmcBlockStatus=1  maskContainerNames=tabcontainer1  block_type=logical  block_config=sysgen:Logical_config
  Logical3 : hdlBasic/Logical  logical_function=AND  inputs=2  en=off  latency=0  precision=Full  arith_type=Unsigned  n_bits=16  bin_pt=0  align_bp=on  overflow=[]  quantization=[]  XmcBlockStatus=1  maskContainerNames=tabcontainer1  block_type=logical  block_config=sysgen:Logical_config
  MCode : hdlBasic/MCode  mfname=CtrlFSM_FFT_MOD  explicit_period=on  period=1/fCIC  iptable={'AXIwrite','';'tlast','';'dcount','';'AXIauto','';'sof',''}  optable={'re','off'}  enable_stdout=off  enable_debug=off  suppress_output=on  defparams={}  hide_port_list={}  block_type=mcode  block_width=444  block_height=788
      settings: infoedit=Pass input values to a MATLAB function for evaluation in Xilinx fixed-point type. The input ports of the block are input arguments of the function. The output ports of the block are output arguments of the function.
  Register{1,3..5} (4 alike) : hdlBasic/Register  init=0  rst=on  en=on  XmcBlockStatus=1  maskContainerNames=tabcontainer1  block_type=register  block_config=sysgen:Register_config
  Relational : hdlBasic/Relational  mode=a>=b  op_type=Bool  en=off  latency=0  XmcBlockStatus=1  maskContainerNames=tabcontainer1  block_type=relational  block_config=sysgen:Relational_config
  Relational1 : hdlBasic/Relational  mode=a<b  op_type=Bool  en=off  latency=0  XmcBlockStatus=1  maskContainerNames=tabcontainer1  block_type=relational  block_config=sysgen:Relational_config
  Terminator : Terminator
  Up Sample1 : hdlBasic/Up Sample  sample_ratio=fCIC/(fHB)  copy_samples=off  en=off  latency=0  XmcBlockStatus=1  maskContainerNames=group1  block_type=usamp  block_config=sysgen:Upsample_config
  Up Sample2 : hdlBasic/Up Sample  sample_ratio=fCIC/(fHB)  copy_samples=off  en=off  latency=0  XmcBlockStatus=1  maskContainerNames=group1  block_type=usamp  block_config=sysgen:Upsample_config
  tdata_out : Outport  VectorParamsAs1DForOutWhenUnconnected=off
  tlast_out : Outport  Port=2  VectorParamsAs1DForOutWhenUnconnected=off
  tvalid_out : Outport  Port=3  VectorParamsAs1DForOutWhenUnconnected=off
  wires:
  Up Sample1/1 -> Register1/1
  Register1/1 -> Convert4/1
  sof/1 -> Up Sample1/1
  Convert4/1 -> MCode/5
  tvalid_in/1 -> FIFO/2
  FIFO/1 -> Register5/1
  Register5/1 -> tdata_out/1
  Convert5/1 -> Logical1/2, Inverter/1, Register4/1
  Register4/1 -> tvalid_out/1
  Register3/1 -> tlast_out/1, Convert1/1
  FIFO/4 -> Relational/1
  auto_restart/1 -> Convert3/1
  Logical3/1 -> Logical2/2
  MCode/1 -> Convert5/1
  packet_size/1 -> Relational1/2
  Constant/1 -> Relational/2
  Relational/1 -> Convert2/1
  Logical/1 -> Counter/1
  Counter/1 -> Relational1/1
  Relational1/1 -> Inverter1/1
  FIFO/3 -> Logical3/1
  tdata_in/1 -> FIFO/1
  Logical1/1 -> Counter/2, Logical2/1
  Inverter1/1 -> Register3/1, Logical/2
  Convert2/1 -> MCode/3
  Convert3/1 -> MCode/4
  tready/1 -> Logical1/1, Register4/3, Register5/3, Register3/3, Register1/3
  Inverter/1 -> Logical3/2
  int_reset/1 -> Up Sample2/1
  transfer/1 -> Convert/1
  Convert/1 -> MCode/1
  Convert1/1 -> MCode/2
  Logical2/1 -> FIFO/3
  FIFO/2 -> Terminator/1
  Up Sample2/1 -> Register4/2, Register3/2, Register5/2, FIFO/4, Logical/1, Register1/2

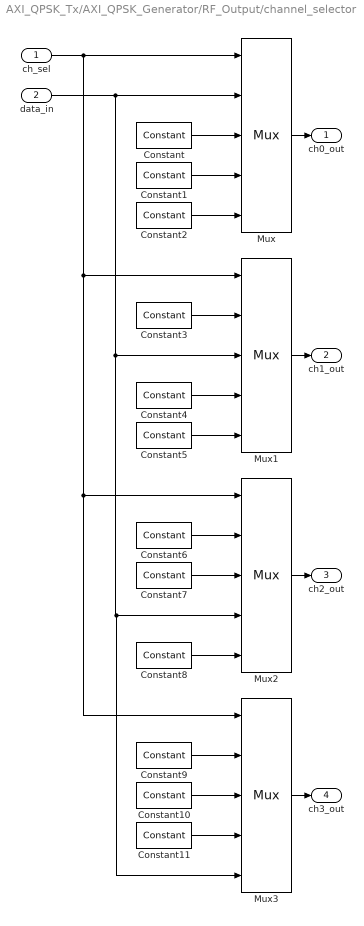
== system AXI_QPSK_Tx/AXI_QPSK_Generator/RF_Output/channel_selector ==
  ch_sel : Inport
  data_in : Inport  Port=2
  Constant{,1..11} (12 alike) : hdlBasic/Constant  const=0  gui_display_data_type=Fixed-point  arith_type=Unsigned  n_bits=32  bin_pt=0  preci_type=Single  exp_width=8  frac_width=24  explicit_period=off  period=1  XmcBlockStatus=1  maskContainerNames=tabcontainer1  block_type=constant  block_config=sysgen:Constant_config
  Mux{,1..3} (4 alike) : hdlBasic/Mux  inputs=4  en=off  latency=1  precision=Full  arith_type=Unsigned  n_bits=16  bin_pt=14  quantization=Truncate  overflow=Wrap  XmcBlockStatus=1  maskContainerNames=tabcontainer1  block_type=mux  block_config=sysgen:Mux_config
  ch0_out : Outport
  ch1_out : Outport  Port=2
  ch2_out : Outport  Port=3
  ch3_out : Outport  Port=4
  wires:
  Constant2/1 -> Mux/5
  Constant7/1 -> Mux2/3
  Constant1/1 -> Mux/4
  Constant11/1 -> Mux3/4
  Constant4/1 -> Mux1/4
  Constant6/1 -> Mux2/2
  Constant/1 -> Mux/3
  Constant5/1 -> Mux1/5
  Constant3/1 -> Mux1/2
  Constant8/1 -> Mux2/5
  Constant10/1 -> Mux3/3
  Constant9/1 -> Mux3/2
  data_in/1 -> Mux3/5, Mux2/4, Mux1/3, Mux/2
  ch_sel/1 -> Mux1/1, Mux2/1, Mux3/1, Mux/1
  Mux2/1 -> ch2_out/1
  Mux/1 -> ch0_out/1
  Mux3/1 -> ch3_out/1
  Mux1/1 -> ch1_out/1

== system AXI_QPSK_Tx/AXI_QPSK_Generator/Symbol_2_Output/M_AXIS_SYMBOL_CTRL ==
  i_data : Inport
  tvalid_in : Inport  Port=2
  q_data : Inport  Port=3
  reset : Inport  Port=4
  packet_size : Inport  Port=5
  tready_in : Inport  Port=6
  transfer : Inport  Port=7
  auto_restart : Inport  Port=8
  AXI_Write_Interface : Subsystem
  Concat : hdlBasic/Concat  num_inputs=2  XmcBlockStatus=1  maskContainerNames=group1  block_type=concat  block_config=sysgen:Concat_config
  Convert4 : hdlBasic/Convert  gui_display_data_type=Fixed-point  arith_type=Unsigned  n_bits=8  bin_pt=0  float_type=Single  exp_bits=8  fraction_bits=24  quantization=Truncate  overflow=Wrap  en=off  latency=0  pipeline=off  XmcBlockStatus=1  maskContainerNames=group2  block_type=convert  block_config=sysgen:Convert_config  block_width=595  block_height=885
  Reinterpret : hdlBasic/Reinterpret  force_arith_type=on  arith_type=Unsigned  force_bin_pt=on  bin_pt=0  XmcBlockStatus=1  maskContainerNames=group1  block_type=reinterpret  block_config=sysgen:Reinterpret_config
  Reinterpret1 : hdlBasic/Reinterpret  force_arith_type=on  arith_type=Unsigned  force_bin_pt=on  bin_pt=0  XmcBlockStatus=1  maskContainerNames=group1  block_type=reinterpret  block_config=sysgen:Reinterpret_config
  tdata_out : Outport  VectorParamsAs1DForOutWhenUnconnected=off
  tvalid_out : Outport  Port=2  VectorParamsAs1DForOutWhenUnconnected=off
  tlast_out : Outport  Port=3  VectorParamsAs1DForOutWhenUnconnected=off
  wires:
  q_data/1 -> Reinterpret/1
  i_data/1 -> Reinterpret1/1
  Reinterpret1/1 -> Concat/2
  Reinterpret/1 -> Concat/1
  packet_size/1 -> AXI_Write_Interface/4(packet_size)
  tvalid_in/1 -> AXI_Write_Interface/6(tvalid_in)
  reset/1 -> AXI_Write_Interface/1(int_reset)
  Concat/1 -> AXI_Write_Interface/5(tdata_in)
  transfer/1 -> AXI_Write_Interface/2(transfer)
  auto_restart/1 -> AXI_Write_Interface/3(auto_restart)
  tready_in/1 -> AXI_Write_Interface/7(tready)
  AXI_Write_Interface/2(tlast_out) -> tlast_out/1
  AXI_Write_Interface/3(tvalid_out) -> tvalid_out/1
  AXI_Write_Interface/1(tdata_out) -> Convert4/1
  Convert4/1 -> tdata_out/1

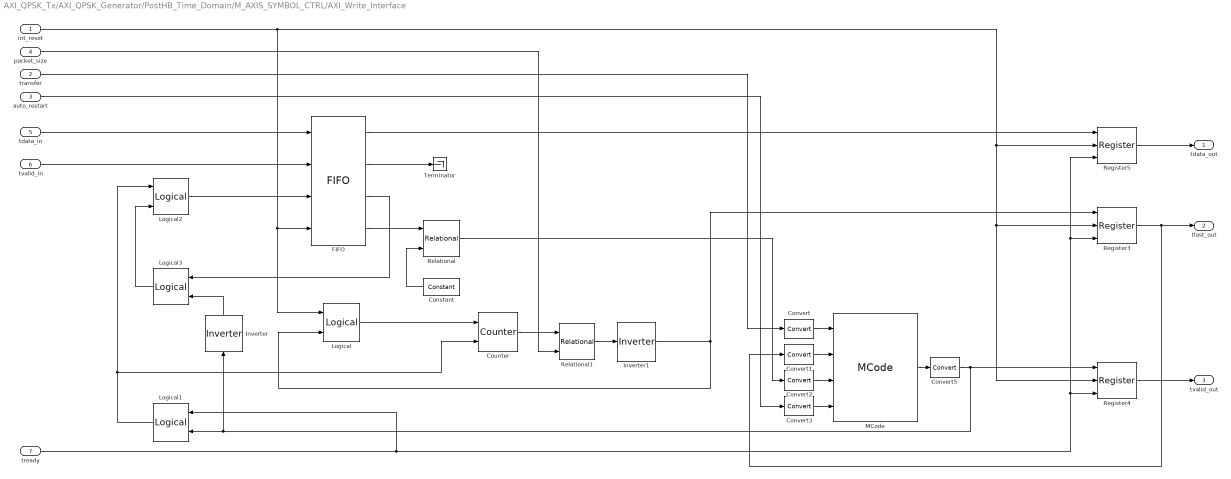
== system AXI_QPSK_Tx/AXI_QPSK_Generator/PostHB_Time_Domain/M_AXIS_SYMBOL_CTRL/AXI_Write_Interface ==
  int_reset : Inport
  transfer : Inport  Port=2
  auto_restart : Inport  Port=3
  packet_size : Inport  Port=4
  tdata_in : Inport  Port=5
  tvalid_in : Inport  Port=6
  tready : Inport  Port=7
  Constant : hdlBasic/Constant  const=2047  gui_display_data_type=Fixed-point  arith_type=Unsigned  n_bits=11  bin_pt=0  preci_type=Single  exp_width=8  frac_width=24  explicit_period=on  period=1/fCIC  XmcBlockStatus=1  maskContainerNames=tabcontainer1  block_type=constant  block_config=sysgen:Constant_config
  Convert{,1..3} (4 alike) : hdlBasic/Convert  gui_display_data_type=Fixed-point  arith_type=Unsigned  n_bits=1  bin_pt=0  float_type=Single  exp_bits=8  fraction_bits=24  quantization=Truncate  overflow=Wrap  en=off  latency=0  pipeline=off  XmcBlockStatus=1  maskContainerNames=group2  block_type=convert  block_config=sysgen:Convert_config  block_width=595  block_height=885
  Convert5 : hdlBasic/Convert  gui_display_data_type=Boolean  arith_type=Boolean  n_bits=1  bin_pt=0  float_type=Single  exp_bits=8  fraction_bits=24  quantization=Truncate  overflow=Wrap  en=off  latency=0  pipeline=off  XmcBlockStatus=1  maskContainerNames=group2  block_type=convert  block_config=sysgen:Convert_config  block_width=595  block_height=885
  Counter : hdlBasic/Counter  cnt_type=Free running  cnt_to=Inf  operation=Up  start_count=0  cnt_by_val=1  arith_type=Unsigned  n_bits=32  bin_pt=0  load_pin=off  rst=on  en=on  explicit_period=Explicit  period=1/fCIC  use_behavioral_HDL=off  implementation=Fabric  XmcBlockStatus=1  maskContainerNames=group1  block_type=counter  block_config=sysgen:Counter_config  block_width=531  block_height=1023
  FIFO : hdlBasic/FIFO  mem_type=Block RAM  performance_options=Standard_FIFO  embedded_registers=off  depth=4K  use_asym_data_widths=off  asym_read_width=32  percent_nbits=1  rst=on  rst_latency=2  en=off  use_dcount=on  use_percent_full_port=off  use_almost_empty=off  almost_empty_thresh=2  use_almost_full=off  use_rd_rst_busy=off  use_wr_rst_busy=off  almost_full_thresh=14  almost_empty_offset=[]  almost_full_offset=[]  explicit_period=off  period=[]  store_only_valid=[]  init_zero=[]  simulation_type=fast_sim  XmcBlockStatus=1  maskContainerNames=tabcontainer1  block_type=fifo  block_config=sysgen:FIFO_config  block_width=538  block_height=997
      settings: infoedit=[]
  Inverter : hdlBasic/Inverter  en=off  latency=0  XmcBlockStatus=1  maskContainerNames=group2  block_type=inv  block_config=sysgen:Inverter_config
  Inverter1 : hdlBasic/Inverter  en=off  latency=0  XmcBlockStatus=1  maskContainerNames=group2  block_type=inv  block_config=sysgen:Inverter_config
  Logical : hdlBasic/Logical  logical_function=OR  inputs=2  en=off  latency=0  precision=Full  arith_type=Unsigned  n_bits=16  bin_pt=0  align_bp=on  overflow=[]  quantization=[]  XmcBlockStatus=1  maskContainerNames=tabcontainer1  block_type=logical  block_config=sysgen:Logical_config
  Logical1 : hdlBasic/Logical  logical_function=AND  inputs=2  en=off  latency=0  precision=Full  arith_type=Unsigned  n_bits=16  bin_pt=0  align_bp=on  overflow=[]  quantization=[]  XmcBlockStatus=1  maskContainerNames=tabcontainer1  block_type=logical  block_config=sysgen:Logical_config
  Logical2 : hdlBasic/Logical  logical_function=OR  inputs=2  en=off  latency=0  precision=Full  arith_type=Unsigned  n_bits=16  bin_pt=0  align_bp=on  overflow=[]  quantization=[]  XmcBlockStatus=1  maskContainerNames=tabcontainer1  block_type=logical  block_config=sysgen:Logical_config
  Logical3 : hdlBasic/Logical  logical_function=AND  inputs=2  en=off  latency=0  precision=Full  arith_type=Unsigned  n_bits=16  bin_pt=0  align_bp=on  overflow=[]  quantization=[]  XmcBlockStatus=1  maskContainerNames=tabcontainer1  block_type=logical  block_config=sysgen:Logical_config
  MCode : hdlBasic/MCode  mfname=CtrlFSM  explicit_period=on  period=1/fCIC  iptable={'AXIwrite','';'tlast','';'dcount','';'AXIauto',''}  optable={'re','off'}  enable_stdout=off  enable_debug=off  suppress_output=on  defparams={}  hide_port_list={}  block_type=mcode  block_width=444  block_height=788
      settings: infoedit=Pass input values to a MATLAB function for evaluation in Xilinx fixed-point type. The input ports of the block are input arguments of the function. The output ports of the block are output arguments of the function.
  Register3 : hdlBasic/Register  init=0  rst=on  en=on  XmcBlockStatus=1  maskContainerNames=tabcontainer1  block_type=register  block_config=sysgen:Register_config
  Register4 : hdlBasic/Register  init=0  rst=on  en=on  XmcBlockStatus=1  maskContainerNames=tabcontainer1  block_type=register  block_config=sysgen:Register_config
  Register5 : hdlBasic/Register  init=0  rst=on  en=on  XmcBlockStatus=1  maskContainerNames=tabcontainer1  block_type=register  block_config=sysgen:Register_config
  Relational : hdlBasic/Relational  mode=a>=b  op_type=Bool  en=off  latency=0  XmcBlockStatus=1  maskContainerNames=tabcontainer1  block_type=relational  block_config=sysgen:Relational_config
  Relational1 : hdlBasic/Relational  mode=a<b  op_type=Bool  en=off  latency=0  XmcBlockStatus=1  maskContainerNames=tabcontainer1  block_type=relational  block_config=sysgen:Relational_config
  Terminator : Terminator
  tdata_out : Outport  VectorParamsAs1DForOutWhenUnconnected=off
  tlast_out : Outport  Port=2  VectorParamsAs1DForOutWhenUnconnected=off
  tvalid_out : Outport  Port=3  VectorParamsAs1DForOutWhenUnconnected=off
  wires:
  Register5/1 -> tdata_out/1
  FIFO/2 -> Terminator/1
  Logical2/1 -> FIFO/3
  Convert1/1 -> MCode/2
  Convert/1 -> MCode/1
  transfer/1 -> Convert/1
  int_reset/1 -> Logical/1, FIFO/4, Register5/2, Register3/2, Register4/2
  Inverter/1 -> Logical3/2
  tready/1 -> Register3/3, Register5/3, Register4/3, Logical1/1
  Convert3/1 -> MCode/4
  Convert2/1 -> MCode/3
  Inverter1/1 -> Logical/2, Register3/1
  Logical1/1 -> Logical2/1, Counter/2
  tdata_in/1 -> FIFO/1
  FIFO/3 -> Logical3/1
  Relational1/1 -> Inverter1/1
  Counter/1 -> Relational1/1
  Logical/1 -> Counter/1
  Relational/1 -> Convert2/1
  Constant/1 -> Relational/2
  packet_size/1 -> Relational1/2
  MCode/1 -> Convert5/1
  Logical3/1 -> Logical2/2
  auto_restart/1 -> Convert3/1
  FIFO/4 -> Relational/1
  Register3/1 -> Convert1/1, tlast_out/1
  Register4/1 -> tvalid_out/1
  Convert5/1 -> Register4/1, Inverter/1, Logical1/2
  FIFO/1 -> Register5/1
  tvalid_in/1 -> FIFO/2

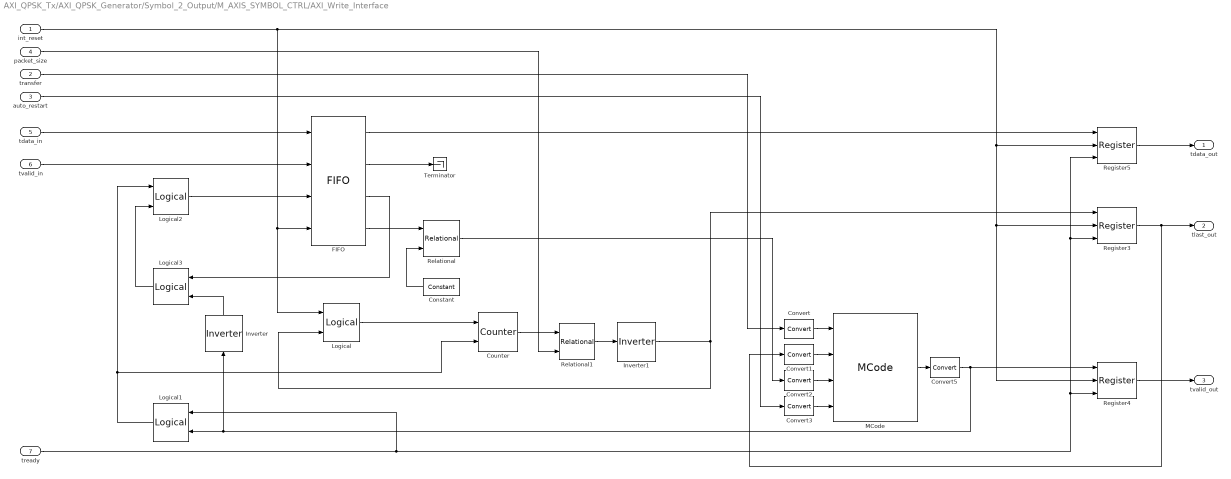
== system AXI_QPSK_Tx/AXI_QPSK_Generator/Symbol_2_Output/M_AXIS_SYMBOL_CTRL/AXI_Write_Interface ==
  int_reset : Inport
  transfer : Inport  Port=2
  auto_restart : Inport  Port=3
  packet_size : Inport  Port=4
  tdata_in : Inport  Port=5
  tvalid_in : Inport  Port=6
  tready : Inport  Port=7
  Constant : hdlBasic/Constant  const=2047  gui_display_data_type=Fixed-point  arith_type=Unsigned  n_bits=11  bin_pt=0  preci_type=Single  exp_width=8  frac_width=24  explicit_period=on  period=1/fCIC  XmcBlockStatus=1  maskContainerNames=tabcontainer1  block_type=constant  block_config=sysgen:Constant_config
  Convert{,1..3} (4 alike) : hdlBasic/Convert  gui_display_data_type=Fixed-point  arith_type=Unsigned  n_bits=1  bin_pt=0  float_type=Single  exp_bits=8  fraction_bits=24  quantization=Truncate  overflow=Wrap  en=off  latency=0  pipeline=off  XmcBlockStatus=1  maskContainerNames=group2  block_type=convert  block_config=sysgen:Convert_config  block_width=595  block_height=885
  Convert5 : hdlBasic/Convert  gui_display_data_type=Boolean  arith_type=Boolean  n_bits=1  bin_pt=0  float_type=Single  exp_bits=8  fraction_bits=24  quantization=Truncate  overflow=Wrap  en=off  latency=0  pipeline=off  XmcBlockStatus=1  maskContainerNames=group2  block_type=convert  block_config=sysgen:Convert_config  block_width=595  block_height=885
  Counter : hdlBasic/Counter  cnt_type=Free running  cnt_to=Inf  operation=Up  start_count=0  cnt_by_val=1  arith_type=Unsigned  n_bits=32  bin_pt=0  load_pin=off  rst=on  en=on  explicit_period=Explicit  period=1/fCIC  use_behavioral_HDL=off  implementation=Fabric  XmcBlockStatus=1  maskContainerNames=group1  block_type=counter  block_config=sysgen:Counter_config  block_width=531  block_height=1023
  FIFO : hdlBasic/FIFO  mem_type=Block RAM  performance_options=Standard_FIFO  embedded_registers=off  depth=4K  use_asym_data_widths=off  asym_read_width=32  percent_nbits=1  rst=on  rst_latency=2  en=off  use_dcount=on  use_percent_full_port=off  use_almost_empty=off  almost_empty_thresh=2  use_almost_full=off  use_rd_rst_busy=off  use_wr_rst_busy=off  almost_full_thresh=14  almost_empty_offset=[]  almost_full_offset=[]  explicit_period=off  period=[]  store_only_valid=[]  init_zero=[]  simulation_type=fast_sim  XmcBlockStatus=1  maskContainerNames=tabcontainer1  block_type=fifo  block_config=sysgen:FIFO_config  block_width=538  block_height=997
      settings: infoedit=[]
  Inverter : hdlBasic/Inverter  en=off  latency=0  XmcBlockStatus=1  maskContainerNames=group2  block_type=inv  block_config=sysgen:Inverter_config
  Inverter1 : hdlBasic/Inverter  en=off  latency=0  XmcBlockStatus=1  maskContainerNames=group2  block_type=inv  block_config=sysgen:Inverter_config
  Logical : hdlBasic/Logical  logical_function=OR  inputs=2  en=off  latency=0  precision=Full  arith_type=Unsigned  n_bits=16  bin_pt=0  align_bp=on  overflow=[]  quantization=[]  XmcBlockStatus=1  maskContainerNames=tabcontainer1  block_type=logical  block_config=sysgen:Logical_config
  Logical1 : hdlBasic/Logical  logical_function=AND  inputs=2  en=off  latency=0  precision=Full  arith_type=Unsigned  n_bits=16  bin_pt=0  align_bp=on  overflow=[]  quantization=[]  XmcBlockStatus=1  maskContainerNames=tabcontainer1  block_type=logical  block_config=sysgen:Logical_config
  Logical2 : hdlBasic/Logical  logical_function=OR  inputs=2  en=off  latency=0  precision=Full  arith_type=Unsigned  n_bits=16  bin_pt=0  align_bp=on  overflow=[]  quantization=[]  XmcBlockStatus=1  maskContainerNames=tabcontainer1  block_type=logical  block_config=sysgen:Logical_config
  Logical3 : hdlBasic/Logical  logical_function=AND  inputs=2  en=off  latency=0  precision=Full  arith_type=Unsigned  n_bits=16  bin_pt=0  align_bp=on  overflow=[]  quantization=[]  XmcBlockStatus=1  maskContainerNames=tabcontainer1  block_type=logical  block_config=sysgen:Logical_config
  MCode : hdlBasic/MCode  mfname=CtrlFSM  explicit_period=on  period=1/fCIC  iptable={'AXIwrite','';'tlast','';'dcount','';'AXIauto',''}  optable={'re','off'}  enable_stdout=off  enable_debug=off  suppress_output=on  defparams={}  hide_port_list={}  block_type=mcode  block_width=444  block_height=788
      settings: infoedit=Pass input values to a MATLAB function for evaluation in Xilinx fixed-point type. The input ports of the block are input arguments of the function. The output ports of the block are output arguments of the function.
  Register3 : hdlBasic/Register  init=0  rst=on  en=on  XmcBlockStatus=1  maskContainerNames=tabcontainer1  block_type=register  block_config=sysgen:Register_config
  Register4 : hdlBasic/Register  init=0  rst=on  en=on  XmcBlockStatus=1  maskContainerNames=tabcontainer1  block_type=register  block_config=sysgen:Register_config
  Register5 : hdlBasic/Register  init=0  rst=on  en=on  XmcBlockStatus=1  maskContainerNames=tabcontainer1  block_type=register  block_config=sysgen:Register_config
  Relational : hdlBasic/Relational  mode=a>=b  op_type=Bool  en=off  latency=0  XmcBlockStatus=1  maskContainerNames=tabcontainer1  block_type=relational  block_config=sysgen:Relational_config
  Relational1 : hdlBasic/Relational  mode=a<b  op_type=Bool  en=off  latency=0  XmcBlockStatus=1  maskContainerNames=tabcontainer1  block_type=relational  block_config=sysgen:Relational_config
  Terminator : Terminator
  tdata_out : Outport  VectorParamsAs1DForOutWhenUnconnected=off
  tlast_out : Outport  Port=2  VectorParamsAs1DForOutWhenUnconnected=off
  tvalid_out : Outport  Port=3  VectorParamsAs1DForOutWhenUnconnected=off
  wires:
  tvalid_in/1 -> FIFO/2
  FIFO/1 -> Register5/1
  Convert5/1 -> Logical1/2, Inverter/1, Register4/1
  Register4/1 -> tvalid_out/1
  Register3/1 -> tlast_out/1, Convert1/1
  FIFO/4 -> Relational/1
  auto_restart/1 -> Convert3/1
  Logical3/1 -> Logical2/2
  MCode/1 -> Convert5/1
  packet_size/1 -> Relational1/2
  Constant/1 -> Relational/2
  Relational/1 -> Convert2/1
  Logical/1 -> Counter/1
  Counter/1 -> Relational1/1
  Relational1/1 -> Inverter1/1
  FIFO/3 -> Logical3/1
  tdata_in/1 -> FIFO/1
  Logical1/1 -> Counter/2, Logical2/1
  Inverter1/1 -> Register3/1, Logical/2
  Convert2/1 -> MCode/3
  Convert3/1 -> MCode/4
  tready/1 -> Logical1/1, Register4/3, Register5/3, Register3/3
  Inverter/1 -> Logical3/2
  int_reset/1 -> Register4/2, Register3/2, Register5/2, FIFO/4, Logical/1
  transfer/1 -> Convert/1
  Convert/1 -> MCode/1
  Convert1/1 -> MCode/2
  Logical2/1 -> FIFO/3
  FIFO/2 -> Terminator/1
  Register5/1 -> tdata_out/1
